simulink model "traj"  (R2017b)
settings: Solver=VariableStepAuto  StartTime=0.0  StopTime=10.0  RelTol=1e-3
values from neighbouring files (symbols this model uses):
  q0 = [pi/12; pi/3; pi/3]    [initial_values.m]
settings Model: Creator=Rita Monteiro  LastModifiedBy=Rita Monteiro

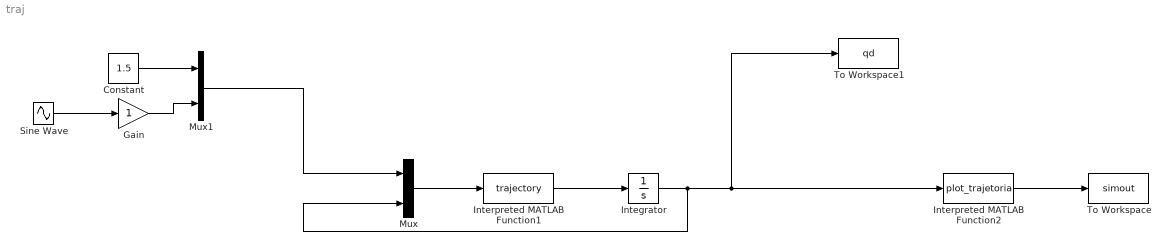
== system traj ==
  Constant : Constant  Value=1.5
  Gain : Gain
  Integrator : Integrator  InitialCondition=q0
  Interpreted MATLAB Function1 : MATLABFcn  MATLABFcn=trajectory
  Interpreted MATLAB Function2 : MATLABFcn  MATLABFcn=plot_trajetoria  OutputDimensions=1
  Mux : Mux  Inputs=2
  Mux1 : Mux  Inputs=2
  Sine Wave : Sin  Frequency=pi/2  Phase=pi/2  SampleTime=0
  To Workspace : ToWorkspace  VariableName=simout  SaveFormat=Timeseries  SampleTime=-1
  To Workspace1 : ToWorkspace  VariableName=qd  SampleTime=-1
  wires:
  Mux/1 -> Interpreted MATLAB Function1/1
  Constant/1 -> Mux1/1
  Interpreted MATLAB Function1/1 -> Integrator/1
  Integrator/1 -> Mux/2, Interpreted MATLAB Function2/1, To Workspace1/1
  Interpreted MATLAB Function2/1 -> To Workspace/1
  Mux1/1 -> Mux/1
  Sine Wave/1 -> Gain/1
  Gain/1 -> Mux1/2
